simulink subsystem "unpack_ToF"  (R2024b)
settings: Solver=VariableStepAuto  StartTime=0.0  StopTime=10.0  RelTol=1e-3
libraries: stmutilitieslib x4
settings Model: Creator=JesseJabezArendse  LastModifiedBy=JesseJabezArendse

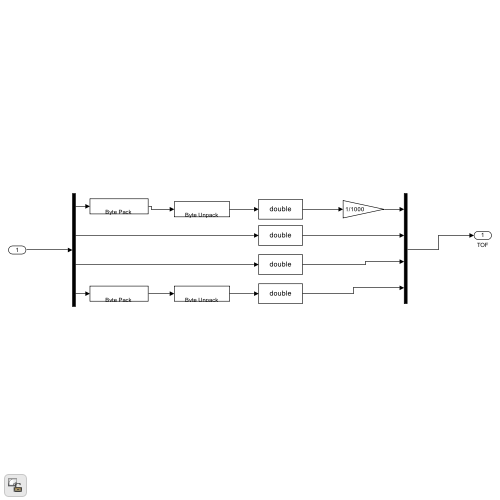
[thumbnail: Simulink's stored preview of the top-level diagram]
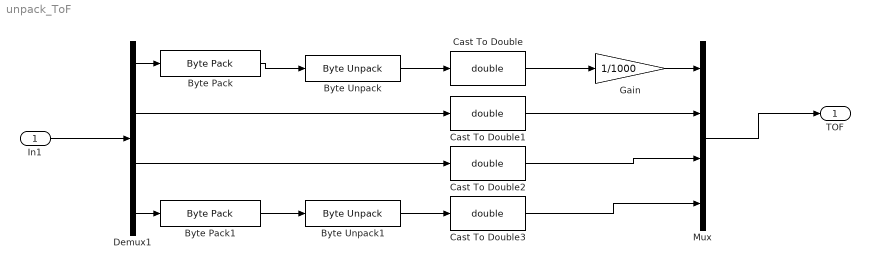
== system unpack_ToF ==
  In1 : Inport
  Byte Pack : stmutilitieslib/Byte Pack  datatypes={'single'}  byteAlign=1  blockPlatform=stm32f4discovery
  Byte Pack1 : stmutilitieslib/Byte Pack  datatypes={'single'}  byteAlign=1  blockPlatform=stm32f4discovery
  Byte Unpack : stmutilitieslib/Byte Unpack  dimensions={[1]}  datatypes={'uint32'}  byteAlign=1  blockPlatform=stm32f4discovery
  Byte Unpack1 : stmutilitieslib/Byte Unpack  dimensions={[1]}  datatypes={'int32'}  byteAlign=1  blockPlatform=stm32f4discovery
  Cast To Double{,1..3} (4 alike) : DataTypeConversion  OutDataTypeStr=double  SaturateOnIntegerOverflow=off  RndMeth=Floor
  Demux1 : Demux
  Gain : Gain  Gain=1/1000
  Mux : Mux
  TOF : Outport
  wires:
  In1/1 -> Demux1/1
  Mux/1 -> TOF/1
  Demux1/2 -> Cast To Double1/1
  Demux1/1 -> Byte Pack/1
  Gain/1 -> Mux/1
  Cast To Double2/1 -> Mux/3
  Byte Unpack/1 -> Cast To Double/1
  Byte Pack/1 -> Byte Unpack/1
  Cast To Double1/1 -> Mux/2
  Demux1/3 -> Cast To Double2/1
  Cast To Double/1 -> Gain/1
  Cast To Double3/1 -> Mux/4
  Byte Pack1/1 -> Byte Unpack1/1
  Byte Unpack1/1 -> Cast To Double3/1
  Demux1/4 -> Byte Pack1/1
